simulink model "Oscilloscopi_offset2020a"  (R2020a)
settings: Solver=FixedStepAuto  StartTime=0.0  StopTime=Inf  RelTol=1e-3
libraries: arduinolib x5, simulink x1
settings Model: SimulationMode=external  ExtModeTrigDuration=2  Creator=Eneko Lerma  LastModifiedBy=FactCore
settings DataIOCC: ReturnWorkspaceOutputs=off
settings OptimizationCC: EnhancedBackFolding=on  PassReuseOutputArgsAs=Individual arguments  MaxStackSize=64  OptimizeBlockOrder=speed  DifferentSizesBufferReuse=on  OptimizationCustomize=off  EfficientTunableParamExpr=on
settings DebuggingCC: ParameterPrecisionLossMsg=none  ParameterTunabilityLossMsg=error  ArithmeticOperatorsInVariantConditions=warning
settings HardwareCC: ProdBitPerPointer=32  ProdBitPerSizeT=32  ProdBitPerPtrDiffT=32  ProdLargestAtomicInteger=Long  ProdLargestAtomicFloat=Double  ProdWordSize=32  ProdHWDeviceType=ARM Compatible->ARM Cortex
settings SFSimCC: SimUseLocalCustomCode=off  MATLABDynamicMemAlloc=off  CustomCodeUndefinedFunction=UseInterfaceOnly
settings RTWCC: SystemTargetFile=ert.tlc  HardwareBoard=Arduino Due  TLCOptions=-aInlineSetEventsForThisBaseRateFcn=TLC_FALSE -aSuppressMultiTaskScheduler=TLC_FALSE -aRateBasedStepFcn=1  TemplateMakefile=ert_default_tmf  GenerateReport=on  RTWUseLocalCustomCode=off  Toolchain=Arduino ARM  BuildConfiguration=Faster Runs  IncludeHyperlinkInReport=on  LaunchReport=on  GenerateTraceInfo=on  GenerateTraceReport=on  GenerateTraceReportSl=on  GenerateTraceReportSf=on  GenerateTraceReportEml=on
settings RTWCC: CustomTerminator=|
  | writeDigitalPin((uint8_T)3, 0);
  | writeDigitalPin((uint8_T)5, 0);
settings CodeAppCC: ForceParamTrailComments=on  IgnoreCustomStorageClasses=off  OperatorAnnotations=on  SimulinkDataObjDesc=on  SFDataObjDesc=on  InsertBlockDesc=on
settings ERTTargetCC: SupportContinuousTime=on  SupportVariableSizeSignals=on

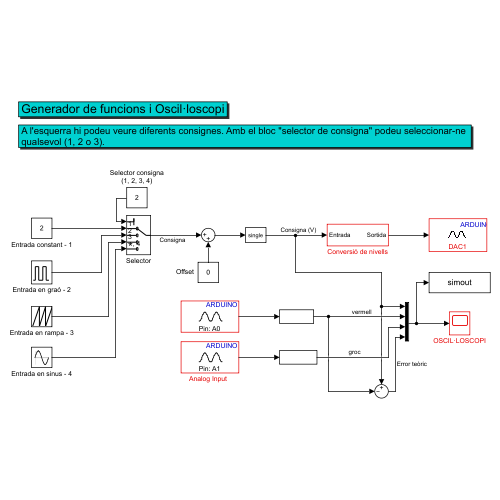
[thumbnail: Simulink's stored preview of the top-level diagram]
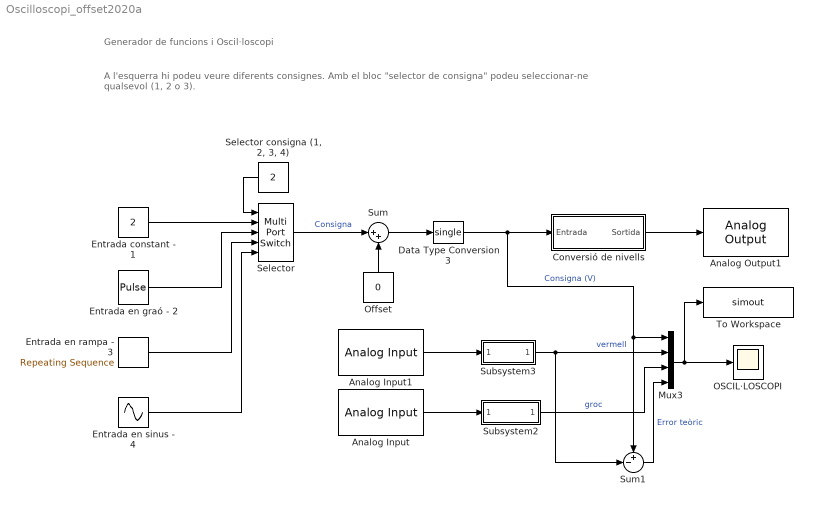
== system Oscilloscopi_offset2020a ==
  note: Generador de funcions i Oscil·loscopi
  note: A l'esquerra hi podeu veure diferents consignes. Amb el bloc "selector de consigna" podeu seleccionar-ne
      | qualsevol (1, 2 o 3).
  "Analog Input  " : arduinolib/Analog Input  pinNumber=1  ReadResultsOnly=off  ConversionTriggerSource=Software  ExternalTriggerType=uint32(0)  OutputDataType=uint16  EnableConversionCompleteNotify=off  EnableOuputStatus=off  SampleTime=0.005  blockPlatform=arduino
  Analog Input1 : arduinolib/Analog Input  pinNumber=0  ReadResultsOnly=off  ConversionTriggerSource=Software  ExternalTriggerType=uint32(0)  OutputDataType=uint16  EnableConversionCompleteNotify=off  EnableOuputStatus=off  SampleTime=0.005  blockPlatform=arduino
  Analog Output1 : arduinolib/Analog Output  DACpin=DAC1  blockPlatform=arduino
      settings: SourceProductBaseCode=ARDUINO
  Conversió de nivells : Subsystem
  Data Type Conversion3 : DataTypeConversion  OutDataTypeStr=single
  Entrada constant - 1 : Constant  Value=2
  Entrada en graó - 2 : DiscretePulseGenerator  PulseType=Time based  Amplitude=2  Period=10  PulseWidth=50
  Entrada en rampa - 3 : simulink/Sources/Repeating Sequence  rep_seq_t=[0 10]  rep_seq_y=[0 0.5]
  Entrada en sinus - 4 : Sin  Amplitude=5  Frequency=2*pi*0.5  SampleTime=0
  Mux3 : Mux
  OSCIL·LOSCOPI : Scope
  Offset : Constant  Value=0
  Selector : MultiPortSwitch  Inputs=4  OutDataTypeStr=single
  "Selector consigna (1, 2, 3, 4)" : Constant  Value=2
  Subsystem2 : Subsystem
  Subsystem3 : Subsystem
  Sum : Sum  Inputs=|++
  Sum1 : Sum  Inputs=+-|
  To Workspace : ToWorkspace  VariableName=simout  SampleTime=-1
  wires:
  Subsystem3/1("   ") -> Mux3/2, Sum1/2  "vermell"
  Subsystem2/1("    ") -> Mux3/3  "groc"
  "Analog Input  "/1 -> Subsystem2/1(" ")
  "Selector consigna (1, 2, 3, 4)"/1 -> Selector/1
  Conversió de nivells/1(Sortida) -> Analog Output1/1
  Analog Input1/1 -> Subsystem3/1("  ")
  Selector/1 -> Sum/1  "Consigna"
  Mux3/1 -> OSCIL·LOSCOPI/1, To Workspace/1
  Data Type Conversion3/1 -> Conversió de nivells/1(Entrada), Mux3/1, Sum1/1  "Consigna (V)"
  Entrada constant - 1/1 -> Selector/2
  Entrada en graó - 2/1 -> Selector/3
  Entrada en rampa - 3/1 -> Selector/4
  Entrada en sinus - 4/1 -> Selector/5
  Offset/1 -> Sum/2
  Sum/1 -> Data Type Conversion3/1
  Sum1/1 -> Mux3/4  "Error teòric"

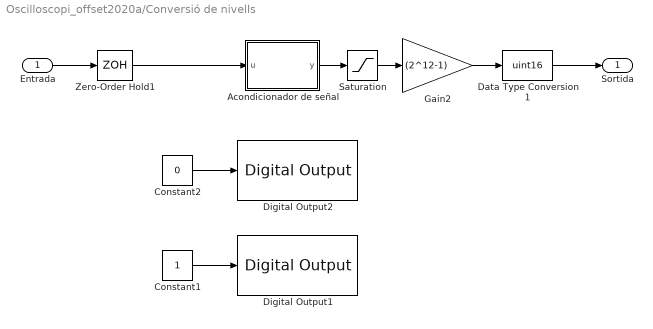
== system Oscilloscopi_offset2020a/Conversió de nivells ==
  Entrada : Inport  OutDataTypeStr=single
  Acondicionador de señal : MATLAB Function  TreatAsAtomicUnit=on
  Constant1 : Constant
  Constant2 : Constant  Value=0
  Data Type Conversion1 : DataTypeConversion  OutDataTypeStr=uint16
  Digital Output1 : arduinolib/Digital Output  pinNumber=5  Direction=output  blockPlatform=arduino
  Digital Output2 : arduinolib/Digital Output  pinNumber=3  Direction=output  blockPlatform=arduino
  Gain2 : Gain  Gain=(2^12-1)  OutDataTypeStr=single
  Saturation : Saturate  UpperLimit=1  LowerLimit=0  OutDataTypeStr=single
  Zero-Order Hold1 : ZeroOrderHold  SampleTime=0.005
  Sortida : Outport  OutDataTypeStr=uint16  VectorParamsAs1DForOutWhenUnconnected=off
  wires:
  Saturation/1 -> Gain2/1
  Data Type Conversion1/1 -> Sortida/1
  Acondicionador de señal/1(y) -> Saturation/1
  Entrada/1 -> Zero-Order Hold1/1
  Gain2/1 -> Data Type Conversion1/1
  Zero-Order Hold1/1 -> Acondicionador de señal/1(u)
  Constant1/1 -> Digital Output1/1
  Constant2/1 -> Digital Output2/1

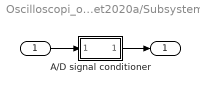
== system Oscilloscopi_offset2020a/Subsystem2 ==
  " " : Inport
  "A/D signal conditioner  " : Subsystem
  "    " : Outport  VectorParamsAs1DForOutWhenUnconnected=off
  wires:
  "A/D signal conditioner  "/1(" ") -> "    "/1
  " "/1 -> "A/D signal conditioner  "/1(" ")

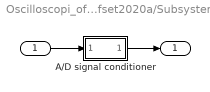
== system Oscilloscopi_offset2020a/Subsystem3 ==
  "  " : Inport
  A/D signal conditioner : Subsystem
  "   " : Outport  VectorParamsAs1DForOutWhenUnconnected=off
  wires:
  A/D signal conditioner/1(" ") -> "   "/1
  "  "/1 -> A/D signal conditioner/1(" ")

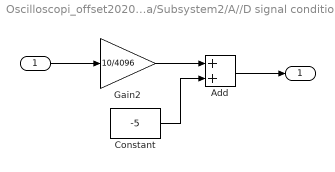
== system Oscilloscopi_offset2020a/Subsystem2/A//D signal conditioner   ==
  " " : Inport
  Add : Sum  AccumDataTypeStr=single
  Constant : Constant  Value=-5  OutDataTypeStr=single
  Gain2 : Gain  Gain=10/4096  OutDataTypeStr=single
  " " : Outport  VectorParamsAs1DForOutWhenUnconnected=off
  wires:
  " "/1 -> Gain2/1
  Constant/1 -> Add/2
  Gain2/1 -> Add/1
  Add/1 -> " "/1

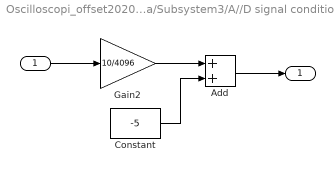
== system Oscilloscopi_offset2020a/Subsystem3/A//D signal conditioner ==
  " " : Inport
  Add : Sum  AccumDataTypeStr=single
  Constant : Constant  Value=-5  OutDataTypeStr=single
  Gain2 : Gain  Gain=10/4096  OutDataTypeStr=single
  " " : Outport  VectorParamsAs1DForOutWhenUnconnected=off
  wires:
  Add/1 -> " "/1
  Gain2/1 -> Add/1
  Constant/1 -> Add/2
  " "/1 -> Gain2/1

== matlab function Oscilloscopi_offset2020a/Conversió de nivells/Acondicionador de señal ==
  data: u input; y output
function y = fcn(u)
y =0.0968*u+0.5058;
